simulink model "Simple_Model_Packaging_6_2"  (R2022b)
settings: Solver=VariableStepAuto  StartTime=0.0  StopTime=0.1  RelTol=1e-3
InitFcn:
  | Parameter_Initialize_6
undefined symbols (not defined in the file or in its folder): gcbh, magnitude, model, rcfiltgaincompat, rsgenpoly
libraries: commdigbbndpm3 x3, commdigbbndam3 x3, commsynccomp2 x3, commblkintrlv2 x2, commfilt2 x2, simulink x2, commblkcod2 x1, commrandsrc3 x1, dspobslib x1, commdigbbndfm2 x1, commseqgen3 x1
settings Model: Creator=89778  LastModifiedBy=z0y

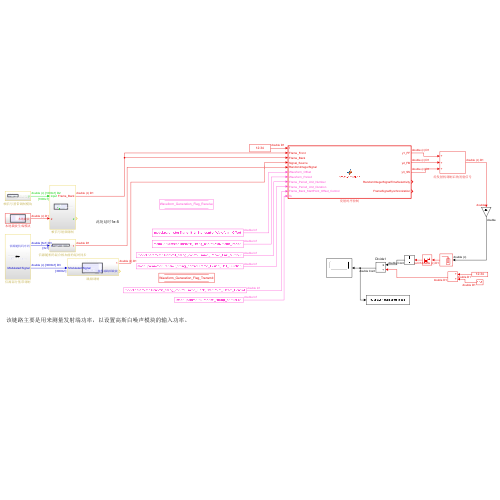
[thumbnail: Simulink's stored preview of the top-level diagram]
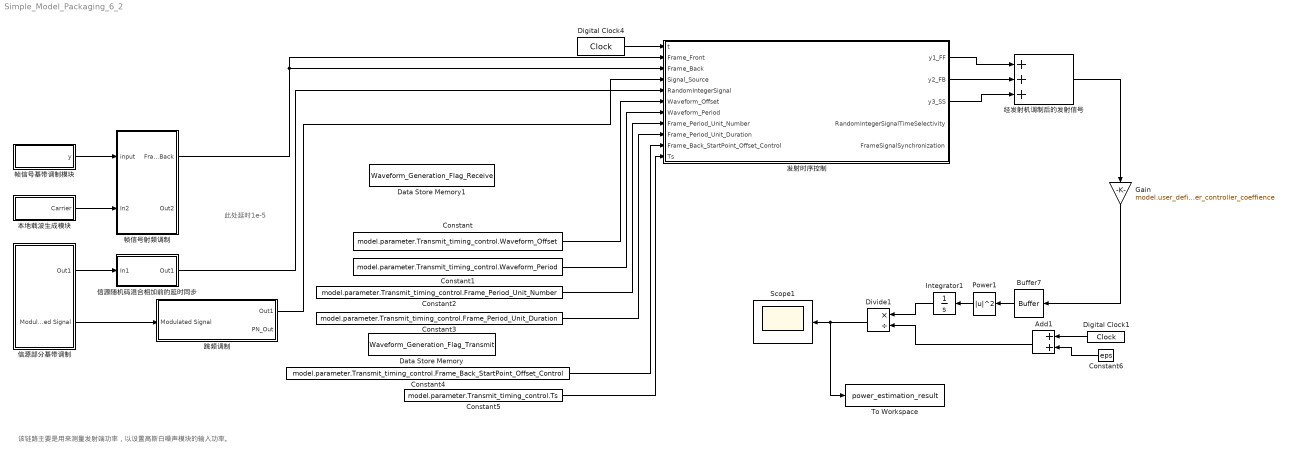
== system Simple_Model_Packaging_6_2 ==
  note: 该链路主要是用来测量发射端功率，以设置高斯白噪声模块的输入功率。
  note: 此处延时1e-5
  Add1 : Sum
  Buffer7 : Buffer  N=1  OutputFrames=off
  Constant : Constant  Value=model.parameter.Transmit_timing_control.Waveform_Offset
  Constant1 : Constant  Value=model.parameter.Transmit_timing_control.Waveform_Period
  Constant2 : Constant  Value=model.parameter.Transmit_timing_control.Frame_Period_Unit_Number
  Constant3 : Constant  Value=model.parameter.Transmit_timing_control.Frame_Period_Unit_Duration
  Constant4 : Constant  Value=model.parameter.Transmit_timing_control.Frame_Back_StartPoint_Offset_Control
  Constant5 : Constant  Value=model.parameter.Transmit_timing_control.Ts
  Constant6 : Constant  Value=eps  SampleTime=model.Intermediate_variable.system_frame_speed_3
  Data Store Memory : DataStoreMemory  DataStoreName=Waveform_Generation_Flag_Transmit  WriteAfterWriteMsg=warning  ShowAdditionalParam=off  OutDataTypeStr=int8
  Data Store Memory1 : DataStoreMemory  DataStoreName=Waveform_Generation_Flag_Receive  WriteAfterWriteMsg=warning  ShowAdditionalParam=off  OutDataTypeStr=int8
  Digital Clock1 : DigitalClock  SampleTime=model.Intermediate_variable.system_frame_speed_3
  Digital Clock4 : DigitalClock  SampleTime=model.parameter.Digital_Clock4.Ts
  Divide1 : Product  Inputs=*/
  Gain : Gain  Gain=model.user_defined.TR.Sig_power_controller_coeffience
  Integrator1 : Integrator
  Power1 : Math  Operator=magnitude^2
  Scope1 : Scope
  To Workspace : ToWorkspace  VariableName=power_estimation_result  SaveFormat=Timeseries  SampleTime=-1
  信源部分基带调制 : Subsystem
  信源随机码混合相加前的延时同步 : Subsystem
  发射时序控制 : MATLAB Function  TreatAsAtomicUnit=on
  帧信号基带调制模块 : Subsystem
  帧信号射频调制 : Subsystem
  本地载波生成模块 : Subsystem
  经发射机调制后的发射信号 : Sum  Inputs=+++
  跳频调制 : Subsystem
  wires:
  帧信号基带调制模块/1(y) -> 帧信号射频调制/1(input)
  本地载波生成模块/1(Carrier) -> 帧信号射频调制/2(In2)
  信源部分基带调制/1(Out1) -> 信源随机码混合相加前的延时同步/1(In1)
  信源部分基带调制/2(Modulated Signal) -> 跳频调制/1(Modulated Signal)
  发射时序控制/3(y3_SS) -> 经发射机调制后的发射信号/3
  发射时序控制/2(y2_FB) -> 经发射机调制后的发射信号/2
  发射时序控制/1(y1_FF) -> 经发射机调制后的发射信号/1
  Constant4/1 -> 发射时序控制/10(Frame_Back_StartPoint_Offset_Control)
  Constant3/1 -> 发射时序控制/9(Frame_Period_Unit_Duration)
  Constant1/1 -> 发射时序控制/7(Waveform_Period)
  信源随机码混合相加前的延时同步/1(Out1) -> 发射时序控制/5(RandomIntegerSignal)
  跳频调制/1(Out1) -> 发射时序控制/4(Signal_Source)
  帧信号射频调制/1(Frame_Back) -> 发射时序控制/3(Frame_Back), 发射时序控制/2(Frame_Front)
  Constant/1 -> 发射时序控制/6(Waveform_Offset)
  Digital Clock4/1 -> 发射时序控制/1(t)
  Constant2/1 -> 发射时序控制/8(Frame_Period_Unit_Number)
  Constant5/1 -> 发射时序控制/11(Ts)
  Add1/1 -> Divide1/2
  Integrator1/1 -> Divide1/1
  Buffer7/1 -> Power1/1
  Divide1/1 -> To Workspace/1, Scope1/1
  Power1/1 -> Integrator1/1
  Digital Clock1/1 -> Add1/1
  经发射机调制后的发射信号/1 -> Gain/1
  Constant6/1 -> Add1/2
  Gain/1 -> Buffer7/1

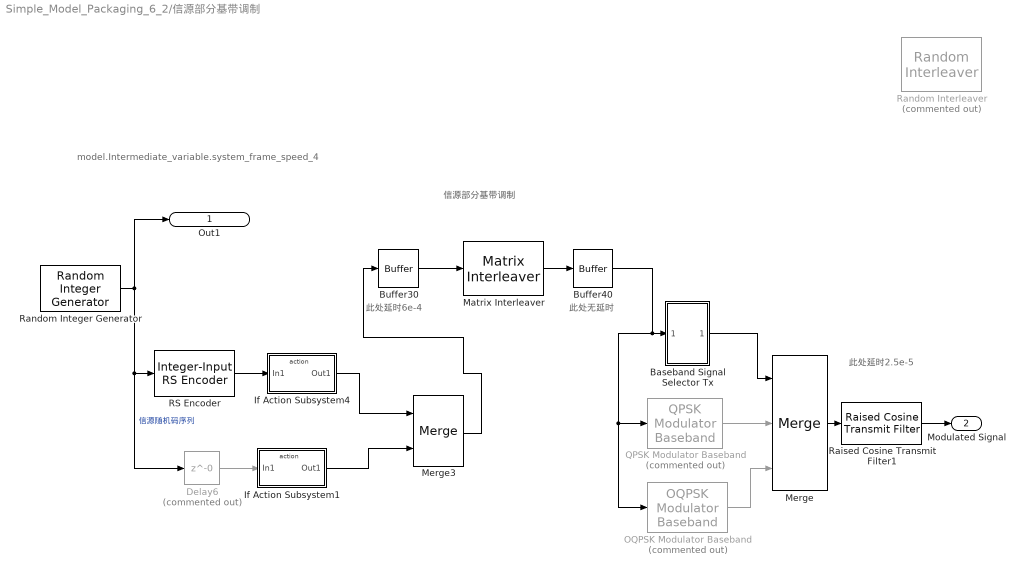
== system Simple_Model_Packaging_6_2/信源部分基带调制 ==
  note: model.Intermediate_variable.system_frame_speed_4
  note: 信源部分基带调制
  note: 此处延时2.5e-5
  note: 此处延时6e-4
  note: 此处无延时
  Baseband Signal Selector Tx : Subsystem
  Buffer30 : Buffer  N=model.parameter.Buffer30.Output_buffer_size  OutputFrames=off
  Buffer40 : Buffer  N=model.parameter.Buffer40.Output_buffer_size  OutputFrames=off
  Delay6 : Delay  Commented=on  DelayLength=0  InitialCondition=0
  If Action Subsystem1 : Subsystem  TreatAsAtomicUnit=on
  If Action Subsystem4 : Subsystem  TreatAsAtomicUnit=on
  Matrix Interleaver : commblkintrlv2/Matrix Interleaver  StatePerturbationForJacobian=1.0e-05  Nrows=model.parameter.Matrix_Interleaver.row_nums  Ncols=model.parameter.Matrix_Interleaver.col_nums
  Merge : Merge  Inputs=3
  Merge3 : Merge
  OQPSK Modulator Baseband : commdigbbndpm3/OQPSK Modulator Baseband  Commented=on  InType=Integer  Ph=0  Mapping=Gray  pulseShape=Half sine  num=[0.7071, 0.7071]  rolloff=0.2  filterSpan=10  sps=2  RateOptions=Enforce single-rate processing  outDtype=double
  QPSK Modulator Baseband : commdigbbndpm3/QPSK Modulator Baseband  Commented=on  InType=Integer  Enc=Gray  Ph=pi/4  outDtype=double  outWordLen=16  outUDDataType=sfix(16)  outFracLenMode=Best precision  outFracLen=15  outDataTypeStr=double  outLastDataTypeStr=double
  RS Encoder : commblkcod2/Integer-Input RS Encoder  n=model.parameter.RS_Encoder.Codeword_length  k=model.parameter.RS_Encoder.Message_length  specShortening=off  shortenedK=3  specGenPoly=off  genPoly=rsgenpoly(7,3)  specPrimPoly=off  prPoly=[1 0 1 1]  specPuncture=off  punctVec=[ones(2,1); zeros(2,1)]
  Raised Cosine Transmit Filter1 : commfilt2/Raised Cosine Transmit Filter  filtType=Square root  R=model.parameter.Raised_Cosine_Transmit_Filter1.Rolloff_factor  filtSpan=model.parameter.Raised_Cosine_Transmit_Filter1.Filter_span_in_symbols  N=model.parameter.Raised_Cosine_Transmit_Filter1.Input_samples_per_symbol  filterGain=rcfiltgaincompat(gcbh)  InputProcessing=Columns as channels (frame based)  RateOptions=Enforce single-rate processing  framing=Mute  checkCoeff=off  variableName=rcTxFilt1  checkGain=Normalized  sampMode=Mute  saveAsFlag=0  currentFiltSpan=10  D=(10)/2  launchFVT=on  roundingMode=Floor  overflowMode=off  coeffDataTypeStr=Inherit: Same word length as input  coeffMin=[]  coeffMax=[]  coeffLastDataTypeStr=Inherit: Same word length as input  outputDataTypeStr=Inherit: Same as accumulator  outputMin=[]  outputMax=[]  outputLastDataTypeStr=Inherit: Same as accumulator
  Random Interleaver : commblkintrlv2/Random Interleaver  Commented=on  StatePerturbationForJacobian=1.0e-05  N=120  seed=12345
  Random Integer Generator : commrandsrc3/Random Integer Generator  SetSize=model.parameter.Random_Integer_Generator.Set_size  SeedSource=Auto  Seed=4  SampleTime=model.parameter.Random_Integer_Generator.SignalSourceTs  SamplesPerFrame=model.parameter.Random_Integer_Generator.Samples_per_frame  OutputDataType=double  SimulateUsing=Interpreted execution
  Out1 : Outport
  Modulated Signal : Outport  Port=2
  wires:
  Raised Cosine Transmit Filter1/1 -> Modulated Signal/1
  Random Integer Generator/1 -> Delay6/1, RS Encoder/1, Out1/1  "信源随机码序列"
  Buffer30/1 -> Matrix Interleaver/1
  Matrix Interleaver/1 -> Buffer40/1
  Merge3/1 -> Buffer30/1
  Baseband Signal Selector Tx/1(Out1) -> Merge/1
  QPSK Modulator Baseband/1 -> Merge/2
  OQPSK Modulator Baseband/1 -> Merge/3
  Buffer40/1 -> QPSK Modulator Baseband/1, OQPSK Modulator Baseband/1, Baseband Signal Selector Tx/1(In1)
  Merge/1 -> Raised Cosine Transmit Filter1/1
  RS Encoder/1 -> If Action Subsystem4/1(In1)
  If Action Subsystem4/1(Out1) -> Merge3/1
  Delay6/1 -> If Action Subsystem1/1(In1)
  If Action Subsystem1/1(Out1) -> Merge3/2

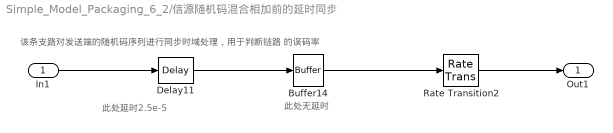
== system Simple_Model_Packaging_6_2/信源随机码混合相加前的延时同步 ==
  note: 此处延时2.5e-5
  note: 该条支路对发送端的随机码序列进行同步时域处理，用于判断链路
      | 的误码率
  note: 此处无延时
  In1 : Inport
  Buffer14 : Buffer  N=model.parameter.Buffer14.Output_buffer_size  OutputFrames=off
  Delay11 : dspobslib/Delay  InputProcessing=Columns as channels (frame based)  dly_unit=Samples  delay=model.parameter.Delay11.samples_length  ic_detail=off  dif_ic_for_ch=on  dif_ic_for_dly=off  ic=0  reset_popup=None
  Rate Transition2 : RateTransition  OutPortSampleTime=model.Intermediate_variable.system_frame_speed_3
  Out1 : Outport
  wires:
  In1/1 -> Delay11/1
  Buffer14/1 -> Rate Transition2/1
  Rate Transition2/1 -> Out1/1
  Delay11/1 -> Buffer14/1

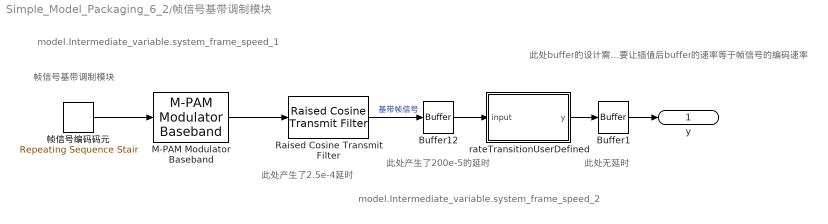
== system Simple_Model_Packaging_6_2/帧信号基带调制模块 ==
  note: model.Intermediate_variable.system_frame_speed_2
  note: model.Intermediate_variable.system_frame_speed_1
  note: 此处buffer的设计需要让插值后buffer的速率等于帧信号的编码速率
  note: 此处产生了200e-5的延时
  note: 帧信号基带调制模块
  note: 此处产生了2.5e-4延时
  note: 此处无延时
  Buffer1 : Buffer  N=model.parameter.Buffer1.Output_buffer_size  OutputFrames=off
  Buffer12 : Buffer  N=model.parameter.Buffer12.Output_buffer_size  OutputFrames=off
  M-PAM Modulator Baseband : commdigbbndam3/M-PAM Modulator Baseband  M=model.parameter.M_PAM_Modulator_Baseband.M_ary_number  InType=Integer  Enc=Gray  PowType=Min. distance between symbols  MinDist=model.parameter.M_PAM_Modulator_Baseband.Minimum_distance  AvgPow=1  PeakPow=1  outDtype=double  outWordLen=16  outUDDataType=sfix(16)  outFracLenMode=Best precision  outFracLen=15  outDataTypeStr=double  outLastDataTypeStr=double
  Raised Cosine Transmit Filter : commfilt2/Raised Cosine Transmit Filter  filtType=Square root  R=model.parameter.Raised_Cosine_Transmit_Filter.Rolloff_factor  filtSpan=model.parameter.Raised_Cosine_Transmit_Filter.Filter_span_in_symbols  N=model.parameter.Raised_Cosine_Transmit_Filter.Output_samples_per_symbol  filterGain=rcfiltgaincompat(gcbh)  InputProcessing=Columns as channels (frame based)  RateOptions=Enforce single-rate processing  framing=Mute  checkCoeff=off  variableName=rcTxFilt  checkGain=Normalized  sampMode=Mute  saveAsFlag=0  currentFiltSpan=10  D=(10)/2  launchFVT=on  roundingMode=Floor  overflowMode=off  coeffDataTypeStr=Inherit: Same word length as input  coeffMin=[]  coeffMax=[]  coeffLastDataTypeStr=Inherit: Same word length as input  outputDataTypeStr=Inherit: Same as accumulator  outputMin=[]  outputMax=[]  outputLastDataTypeStr=Inherit: Same as accumulator
  rateTransitionUserDefined : MATLAB Function  TreatAsAtomicUnit=on
  帧信号编码码元 : simulink/Sources/Repeating Sequence Stair  OutValues=model.parameter.Repeating_Sequence_Stair.output_vector  tsamp=model.parameter.Repeating_Sequence_Stair.CodeTs  OutMin=[]  OutMax=[]  OutDataTypeStr=double  OutputDataTypeScalingMode=double  OutDataType=fixdt(0,8)  ConRadixGroup=Best Precision: Vector-wise  OutScaling=2^-12
  y : Outport
  wires:
  帧信号编码码元/1 -> M-PAM Modulator Baseband/1
  M-PAM Modulator Baseband/1 -> Raised Cosine Transmit Filter/1
  Raised Cosine Transmit Filter/1 -> Buffer12/1  "基带帧信号"
  rateTransitionUserDefined/1(y) -> Buffer1/1
  Buffer1/1 -> y/1
  Buffer12/1 -> rateTransitionUserDefined/1(input)

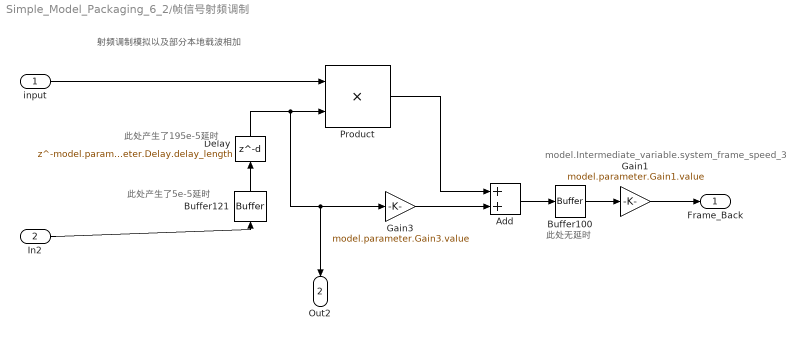
== system Simple_Model_Packaging_6_2/帧信号射频调制 ==
  note: model.Intermediate_variable.system_frame_speed_3
  note: 此处无延时
  note: 此处产生了5e-5延时
  note: 射频调制模拟以及部分本地载波相加
  note: 此处产生了195e-5延时
  input : Inport
  In2 : Inport  Port=2
  Add : Sum
  Buffer100 : Buffer  N=model.parameter.Buffer100.Output_buffer_size  OutputFrames=off
  Buffer121 : Buffer  N=model.parameter.Buffer121.Output_buffer_size  OutputFrames=off
  Delay : Delay  DelayLength=model.parameter.Delay.delay_length  InputProcessing=Columns as channels (frame based)
  Gain1 : Gain  Gain=model.parameter.Gain1.value
  Gain3 : Gain  Gain=model.parameter.Gain3.value
  Product : Product
  Frame_Back : Outport
  Out2 : Outport  Port=2
  wires:
  In2/1 -> Buffer121/1
  Product/1 -> Add/1
  Gain3/1 -> Add/2
  Buffer121/1 -> Delay/1
  Add/1 -> Buffer100/1
  Buffer100/1 -> Gain1/1
  input/1 -> Product/1
  Delay/1 -> Gain3/1, Out2/1, Product/2
  Gain1/1 -> Frame_Back/1

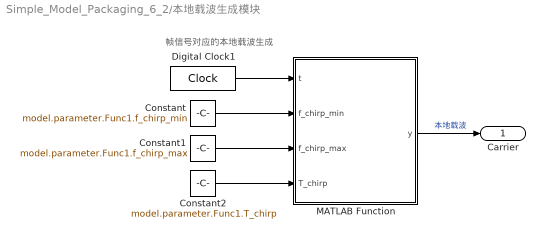
== system Simple_Model_Packaging_6_2/本地载波生成模块 ==
  note: 帧信号对应的本地载波生成
  Constant : Constant  Value=model.parameter.Func1.f_chirp_min
  Constant1 : Constant  Value=model.parameter.Func1.f_chirp_max
  Constant2 : Constant  Value=model.parameter.Func1.T_chirp
  Digital Clock1 : DigitalClock  SampleTime=model.parameter.Digital_Clock2.CarrierTs
  MATLAB Function : MATLAB Function  TreatAsAtomicUnit=on
  Carrier : Outport
  wires:
  Digital Clock1/1 -> MATLAB Function/1(t)
  MATLAB Function/1(y) -> Carrier/1  "本地载波"
  Constant/1 -> MATLAB Function/2(f_chirp_min)
  Constant1/1 -> MATLAB Function/3(f_chirp_max)
  Constant2/1 -> MATLAB Function/4(T_chirp)

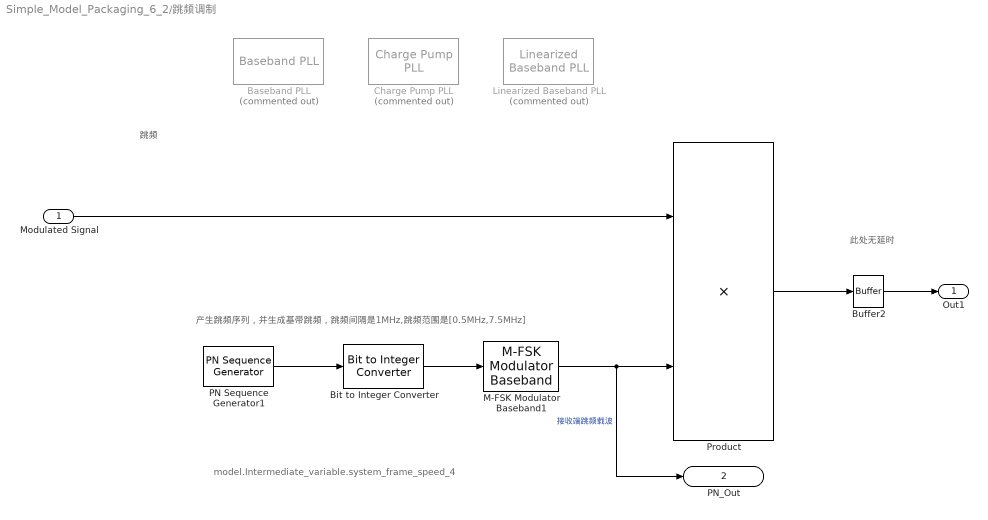
== system Simple_Model_Packaging_6_2/跳频调制 ==
  note: model.Intermediate_variable.system_frame_speed_4
  note: 跳频
  note: 此处无延时
  note: 产生跳频序列，并生成基带跳频，跳频间隔是1MHz,跳频范围是[0.5MHz,7.5MHz]
  Modulated Signal : Inport
  Baseband PLL : commsynccomp2/Baseband PLL  Commented=on  Fn="[3.0002  0  40002]"  Fd="[1   67.46   2270.9   40002]"  Kvco=1
  Bit to Integer Converter : simulink/Logic and Bit Operations/Bit to Integer Converter  nbits=model.parameter.Bit_to_Integer_Converter.M  bitOrder=MSB first  signedOutputValues=Unsigned  outDtype=double  outDtypeSigned=Inherit via internal rule
  Buffer2 : Buffer  N=model.parameter.Buffer2.Output_buffer_size  OutputFrames=off
  Charge Pump PLL : commsynccomp2/Charge Pump PLL  Commented=on  Fn="[3.0002  0  40002]"  Fd="[1   67.46   2270.9   40002]"  Kvco=1  Fc=100  Ph=0  Ac=1
  Linearized Baseband PLL : commsynccomp2/Linearized Baseband PLL  Commented=on  Fn="[3.0002  0  40002]"  Fd="[1   67.46   2270.9   40002]"  Kvco=1
  M-FSK Modulator Baseband1 : commdigbbndfm2/M-FSK Modulator Baseband  M=model.parameter.M_FSK_Modulator_Baseband1.M_ary_number  InType=Integer  Enc=Gray  freqSep=model.parameter.M_FSK_Modulator_Baseband1.Frequency_separation  phaseType=Continuous  numSamp=model.parameter.M_FSK_Modulator_Baseband1.Samples_per_symbol  RateOptions=Enforce single-rate processing  outDataType=double
  PN Sequence Generator1 : commseqgen3/PN Sequence Generator  poly=model.parameter.PN_Sequence_Generator1.Generator_polynomial  ini_sta=model.parameter.PN_Sequence_Generator1.Initial_states  outBitMaskSource=Dialog parameter  shift=0  outVarSiz=off  maxOutSizeMode=Dialog parameter  maxOutSize=[10 1]  Ts=model.parameter.PN_Sequence_Generator1.Sample_time  sampPerFrame=model.parameter.PN_Sequence_Generator1.Samples_per_frame  reset=off  bitPackedOutputs=off  outDataType=double  numPackedBits=5  bitPackDataSigned=off  bitPackedOutDType=double
  Product : Product
  Out1 : Outport
  PN_Out : Outport  Port=2
  wires:
  M-FSK Modulator Baseband1/1 -> PN_Out/1, Product/2  "接收端跳频载波"
  Product/1 -> Buffer2/1
  Buffer2/1 -> Out1/1
  Modulated Signal/1 -> Product/1
  PN Sequence Generator1/1 -> Bit to Integer Converter/1
  Bit to Integer Converter/1 -> M-FSK Modulator Baseband1/1

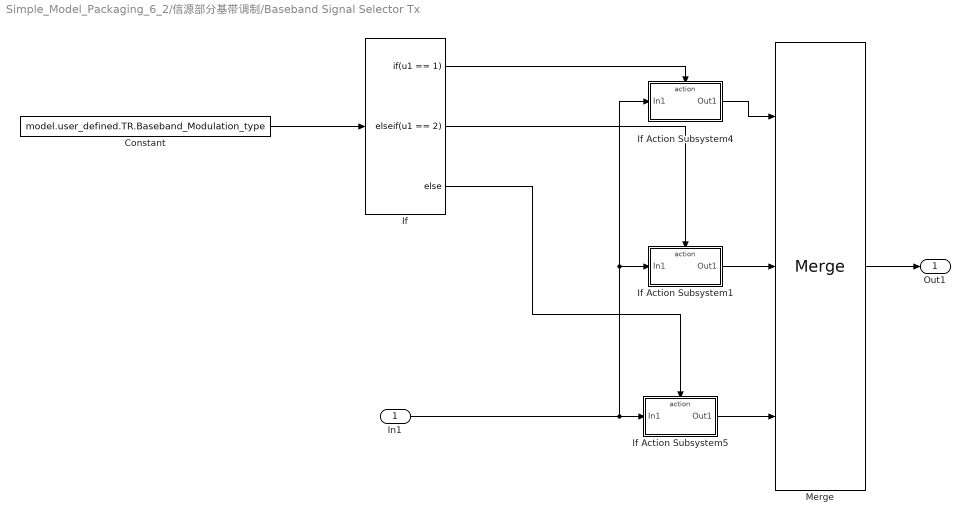
== system Simple_Model_Packaging_6_2/信源部分基带调制/Baseband Signal Selector Tx ==
  In1 : Inport
  Constant : Constant  Value=model.user_defined.TR.Baseband_Modulation_type
  If : If  IfExpression=u1 == 1  ElseIfExpressions=u1 == 2
  If Action Subsystem1 : Subsystem  TreatAsAtomicUnit=on
  If Action Subsystem4 : Subsystem  TreatAsAtomicUnit=on
  If Action Subsystem5 : Subsystem  TreatAsAtomicUnit=on
  Merge : Merge  Inputs=3
  Out1 : Outport
  wires:
  If Action Subsystem5/1(Out1) -> Merge/3
  Constant/1 -> If/1
  Merge/1 -> Out1/1
  If/3 -> If Action Subsystem5/Action
  If/1 -> If Action Subsystem4/Action
  If/2 -> If Action Subsystem1/Action
  If Action Subsystem1/1(Out1) -> Merge/2
  If Action Subsystem4/1(Out1) -> Merge/1
  In1/1 -> If Action Subsystem4/1(In1), If Action Subsystem1/1(In1), If Action Subsystem5/1(In1)

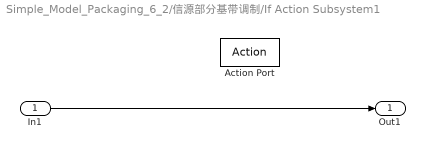
== system Simple_Model_Packaging_6_2/信源部分基带调制/If Action Subsystem1 ==
  In1 : Inport
  Action Port : ActionPort
  Out1 : Outport
  wires:
  In1/1 -> Out1/1

== system Simple_Model_Packaging_6_2/信源部分基带调制/If Action Subsystem4 ==
  In1 : Inport
  Action Port : ActionPort
  Out1 : Outport
  wires:
  In1/1 -> Out1/1

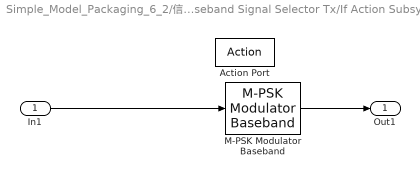
== system Simple_Model_Packaging_6_2/信源部分基带调制/Baseband Signal Selector Tx/If Action Subsystem1 ==
  In1 : Inport
  Action Port : ActionPort  ActionPortLabel=elseif(u1 == 2)
  M-PSK Modulator Baseband : commdigbbndpm3/M-PSK Modulator Baseband  M=model.user_defined.Rectangular_QAM_Modulator_Baseband.M_Number  InType=Integer  Enc=Gray  Mapping=[0:7]  Ph=0  outDtype=double  outWordLen=16  outUDDataType=sfix(16)  outFracLenMode=Best precision  outFracLen=15  outDataTypeStr=double  outLastDataTypeStr=double
  Out1 : Outport
  wires:
  M-PSK Modulator Baseband/1 -> Out1/1
  In1/1 -> M-PSK Modulator Baseband/1

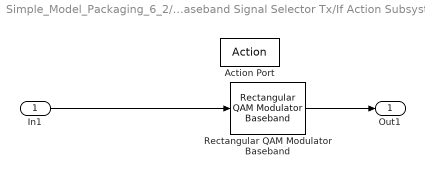
== system Simple_Model_Packaging_6_2/信源部分基带调制/Baseband Signal Selector Tx/If Action Subsystem4 ==
  In1 : Inport
  Action Port : ActionPort  ActionPortLabel=if(u1 == 1)
  Rectangular QAM Modulator Baseband : commdigbbndam3/Rectangular QAM Modulator Baseband  M=model.user_defined.Rectangular_QAM_Modulator_Baseband.M_Number  InType=Integer  Enc=Gray  Mapping=[0:15]  PowType=Min. distance between symbols  MinDist=model.parameter.Rectangular_QAM_Modulator_Baseband.Minimum_distance  AvgPow=1  PeakPow=1  Ph=0  outDtype=double  outWordLen=16  outUDDataType=sfix(16)  outFracLenMode=Best precision  outFracLen=15  outDataTypeStr=double  outLastDataTypeStr=double
      settings: LibrarySourceBlock=|
      | commhdldigbbndam/Rectangular QAM
      | Modulator
      | Baseband
  Out1 : Outport
  wires:
  Rectangular QAM Modulator Baseband/1 -> Out1/1
  In1/1 -> Rectangular QAM Modulator Baseband/1

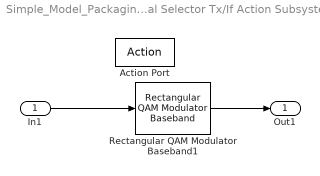
== system Simple_Model_Packaging_6_2/信源部分基带调制/Baseband Signal Selector Tx/If Action Subsystem5 ==
  In1 : Inport
  Action Port : ActionPort  ActionPortLabel=else
  Rectangular QAM Modulator Baseband1 : commdigbbndam3/Rectangular QAM Modulator Baseband  M=model.user_defined.Rectangular_QAM_Modulator_Baseband.M_Number  InType=Integer  Enc=Gray  Mapping=[0:15]  PowType=Min. distance between symbols  MinDist=2  AvgPow=1  PeakPow=1  Ph=0  outDtype=double  outWordLen=16  outUDDataType=sfix(16)  outFracLenMode=Best precision  outFracLen=15  outDataTypeStr=double  outLastDataTypeStr=double
      settings: LibrarySourceBlock=|
      | commhdldigbbndam/Rectangular QAM
      | Modulator
      | Baseband
  Out1 : Outport
  wires:
  In1/1 -> Rectangular QAM Modulator Baseband1/1
  Rectangular QAM Modulator Baseband1/1 -> Out1/1

== matlab function Simple_Model_Packaging_6_2/本地载波生成模块/MATLAB Function ==
  data: y output; t input; f_chirp_min input; f_chirp_max input; T_chirp input
% function y = carrierGenerator(t)
%     fc = 5e6;
%     y = exp(1i*2*pi*fc*t);

function y = carrierGenerator(t, f_chirp_min, f_chirp_max, T_chirp)
    k_chirp = (f_chirp_max-f_chirp_min)/T_chirp;
    t = mod(t,T_chirp);
    y = exp(1i*2*pi*(f_chirp_min*t+0.5*k_chirp*t^2));

end

== matlab function Simple_Model_Packaging_6_2/发射时序控制 ==
  data: t input; y1_FF output; Frame_Front input; Waveform_Generation_Flag_Transmit data_store_memory; Frame_Back input; y2_FB output; y3_SS output; Signal_Source input; RandomIntegerSignal input; RandomIntegerSignalTimeSelectivity output; FrameSignalSynchronization output; Waveform_Offset input; Waveform_Period input; Frame_Period_Unit_Number input; Frame_Period_Unit_Duration input; Frame_Back_StartPoint_Offset_Control input; Ts input
function [y1_FF, y2_FB, y3_SS, RandomIntegerSignalTimeSelectivity, FrameSignalSynchronization] = timeController(t, Frame_Front, Frame_Back, Signal_Source, RandomIntegerSignal, Waveform_Offset, Waveform_Period, Frame_Period_Unit_Number, Frame_Period_Unit_Duration, Frame_Back_StartPoint_Offset_Control, Ts)
global Waveform_Generation_Flag_Transmit;

Frame_Duration = Frame_Period_Unit_Duration * Frame_Period_Unit_Number;
Frame_Front_StartPoint = mod(t-Waveform_Offset, Waveform_Period);
Frame_Back_StartPoint = mod(t-Waveform_Offset, Waveform_Period) - (Waveform_Period - Frame_Duration - Frame_Back_StartPoint_Offset_Control);
Signal_Source_StartPoint = Frame_Front_StartPoint + Frame_Duration;
Signal_Source_EndPoint = Frame_Back_StartPoint;
Frame_Back_EndPoint = Frame_Back_StartPoint - Frame_Duration;

% global Waveform_Generation_Flag;

% if  ( Frame_Front_StartPoint < Ts/10) || ((Frame_Back_StartPoint > -Ts/10) && (Frame_Back_StartPoint < Ts/10)) || ((Signal_Source_StartPoint>-Ts/10) && (Signal_Source_EndPoint<Ts/10))
if  ( Frame_Front_StartPoint < Ts/100) || ((Frame_Back_StartPoint > -Ts/100) && (Frame_Back_EndPoint < Ts/100)) || ((Signal_Source_StartPoint>-Ts/100) && (Signal_Source_EndPoint<Ts/100))
    Waveform_Generation_Flag_Transmit = int8(1);
end

if Waveform_Generation_Flag_Transmit == int8(1)
    if Frame_Front_StartPoint < Frame_Duration
        y1_FF = Frame_Front;
        y2_FB = complex(0);
        y3_SS = complex(0);
        RandomIntegerSignalTimeSelectivity = 0;
        FrameSignalSynchronization = 0;

    elseif (Frame_Back_StartPoint>=0) && (Frame_Back_StartPoint<Frame_Duration)
        y1_FF = complex(0);
        y2_FB = Frame_Back;
        y3_SS = complex(0);
        RandomIntegerSignalTimeSelectivity = 0;
        FrameSignalSynchronization = 0;

    elseif (Signal_Source_StartPoint>0) && (Signal_Source_EndPoint<0)
        y1_FF = complex(0);
        y2_FB = complex(0);
        y3_SS = Signal_Source;
        RandomIntegerSignalTimeSelectivity = RandomIntegerSignal;
        FrameSignalSynchronization = 1;
    else
        Waveform_Generation_Flag_Transmit = int8(0);
        y1_FF = complex(0);
        y2_FB = complex(0);
        y3_SS = complex(0);
        RandomIntegerSignalTimeSelectivity = 0;
        FrameSignalSynchronization = 0;
    end
else
    y1_FF = complex(0);
    y2_FB = complex(0);
    y3_SS = complex(0);
    RandomIntegerSignalTimeSelectivity = 0;
    FrameSignalSynchronization = 0;
end


end

== matlab function Simple_Model_Packaging_6_2/帧信号基带调制模块/rateTransitionUserDefined ==
  data: y output; input input
% function y = carrierGenerator(t)
%     fc = 5e6;
%     y = exp(1i*2*pi*fc*t);

function y = rateTransition(input)
    p = 10;
    q = 1;
    y = resample(input,p,q);
%     y(1:100) = repmat(y(100),1,100);
%     y(end-99:end) = repmat(y(end-99),1,100);
end
